simulink model "invPendModel"  (R2022a)
settings: Solver=VariableStepAuto  StartTime=0.0  StopTime=10.0  RelTol=1e-3
values from neighbouring files (symbols this model uses):
  Ac = (A-B*K)    [pendulum_setup.m]
  inv_pendulum_ss = ss(A,B,C,D,'statename',states,'inputname',inputs,'outputname',outputs)    [pendulum_setup.m]
settings Model: Creator=aakashramachandran  LastModifiedBy=aakashramachandran

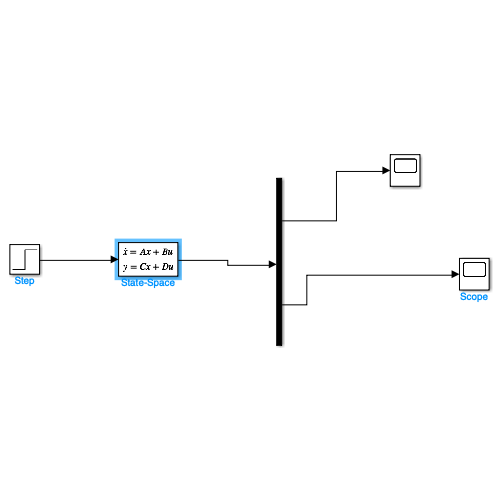
[thumbnail: Simulink's stored preview of the top-level diagram]
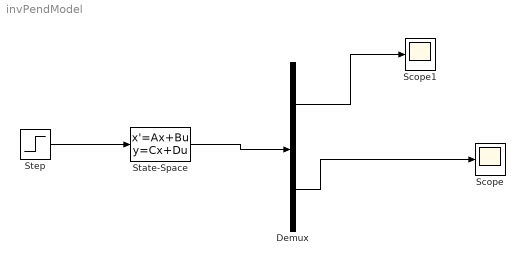
== system invPendModel ==
  Demux : Demux  Outputs=2
  Scope : Scope
  Scope1 : Scope
  State-Space : StateSpace  A=Ac  B=inv_pendulum_ss.B  C=inv_pendulum_ss.C  D=inv_pendulum_ss.D  InitialCondition=[0, 0, 0, 0]  ContinuousStateAttributes={'x' 'x_dot' 'theta' 'theta_dot'};
  Step : Step  Time=0  After=0.2  SampleTime=0
  wires:
  State-Space/1 -> Demux/1
  Demux/2 -> Scope/1
  Step/1 -> State-Space/1
  Demux/1 -> Scope1/1
